simulink model "sf_pw_if_"  (Simulink 7.4)
settings: Solver=FixedStepDiscrete  StartTime=0.0  StopTime=10.0  RelTol=1e-3
settings Model: Creator=vreddy  LastModifiedBy=rcobbe
settings ConfigSet: Description=Default Configuration
settings OptimizationCC: InlineParams=on  InlineInvariantSignals=on  StateBitsets=on  DataBitsets=on  UseTempVars=on  ZeroExternalMemoryAtStartup=off  ZeroInternalMemoryAtStartup=off  NoFixptDivByZeroProtection=on  EfficientFloat2IntCast=on  OptimizeModelRefInitCode=on  LifeSpan=1
settings DebuggingCC: SignalInfNanChecking=warning  SaveWithParameterizedLinksMsg=none
settings RTWCC: SystemTargetFile=ert.tlc  TemplateMakefile=ert_default_tmf  Description=Real-Time Workshop Embedded Coder (no auto configuration)  ProcessScript=ert_make_rtw_hook
settings CodeAppCC: IgnoreCustomStorageClasses=off
settings ERTTargetCC: TargetFcnLib=ansi_tfl_tmw.mat  MultiwordLength=2048  GenerateSampleERTMain=on  InlinedParameterPlacement=NonHierarchical  ERTCustomFileTemplate=example_file_process.tlc  ConvertIfToSwitch=off

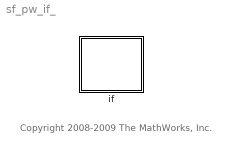
== system sf_pw_if_ ==
  note: Copyright 2008-2009 The MathWorks, Inc.
  if : Stateflow chart

== stateflow chart if ==
  (junction 7) -> (junction 3)
  (junction 6) -> (junction 7) [order 2]
  (junction 4) -> (junction 7)
  (junction 5) -> (junction 4) : {action1}
  (junction 6) -> (junction 5) [order 1] : [condition1]
  (default) -> (junction 6) : /*comment*/
